simulink model "do_sada"  (R2016b)
settings: Solver=VariableStepAuto  StartTime=0.0  StopTime=10000.0  RelTol=1e-12  AbsTol=1e-9
values from neighbouring files (symbols this model uses):
  d1 = 0.0012    [main.m]
  d2 = 0.0012    [main.m]
  d3 = 0.0012    [main.m]
  h0 = 3    [main.m]
  h10 = 4    [main.m]
  h20 = 4    [main.m]
  h30 = 4    [main.m]
  hmax = 10    [main.m]
  K = acker(Al, Bl, P)    [main.m]
  kr = -1/(Cl * ((Al-Bl*K)\Bl))    [main.m]
  q0 = A * sqrt(h0) / B    [main.m]
  r = 3    [main.m]
  s = 1    [main.m]
  sout = 10e-4    (= 0.001)    [main.m]
settings Model: Creator=Vukan  LastModifiedBy=Vukan

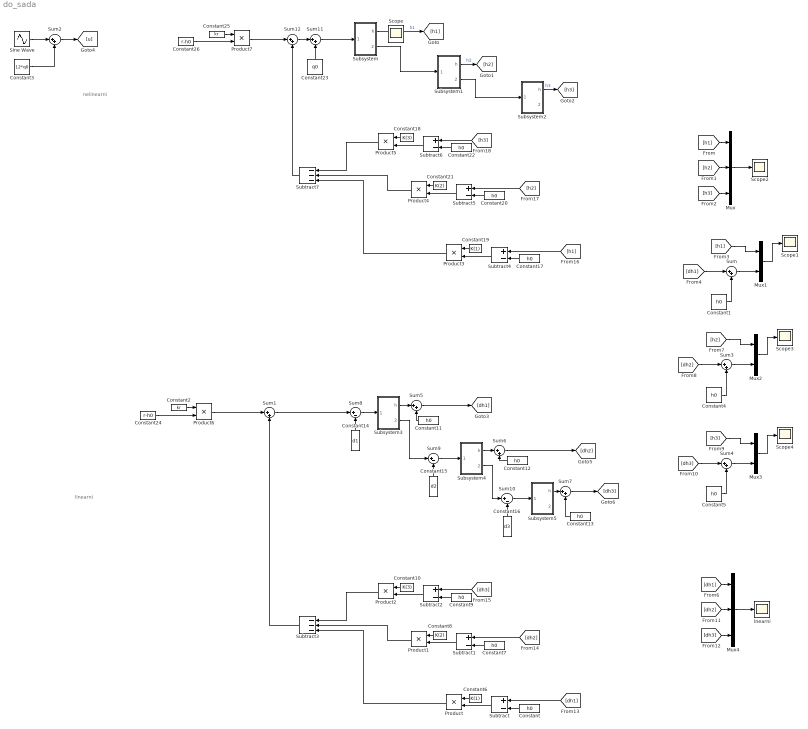
== system do_sada ==
  note: nelinearni
  note: linearni
  Constant{,1,4..5,7,9,11..13,17,20,22} (12 alike) : Constant  Value=h0
  Constant10 : Constant  Value=K(3)
  Constant14 : Constant  Value=d1
  Constant15 : Constant  Value=d2
  Constant16 : Constant  Value=d3
  Constant18 : Constant  Value=K(3)
  Constant19 : Constant  Value=K(1)
  Constant2 : Constant  Value=kr
  Constant21 : Constant  Value=K(2)
  Constant23 : Constant  Value=q0
  Constant24 : Constant  Value=r-h0
  Constant25 : Constant  Value=kr
  Constant26 : Constant  Value=r-h0
  Constant3 : Constant  Value=12*q0
  Constant6 : Constant  Value=K(1)
  Constant8 : Constant  Value=K(2)
  Mux : Mux  Inputs=3
  Mux1 : Mux  Inputs=2
  Mux2 : Mux  Inputs=2
  Mux3 : Mux  Inputs=2
  Mux4 : Mux  Inputs=3
  Product{,1..7} (8 alike) : Product
  Scope{,1..4} (5 alike) : Scope
  Sine Wave : Sin  Amplitude=10*q0  Frequency=0.001*30  SampleTime=0
  Subsystem : Subsystem
  Subsystem1 : Subsystem
  Subsystem2 : Subsystem
  Subsystem3 : Subsystem
  Subsystem4 : Subsystem
  Subsystem5 : Subsystem
  Subtract{,1..2,4..6} (6 alike) : Sum  Inputs=+-
  Subtract3 : Sum  Inputs=---
  Subtract7 : Sum  Inputs=---
  Sum{,1..7,11..12} (10 alike) : Sum  Inputs=|++
  Sum10 : Sum  Inputs=|+-
  Sum8 : Sum  Inputs=|+-
  Sum9 : Sum  Inputs=|+-
  lnearni : Scope
  wires:
  Subsystem/1(h) -> [h1]  "h1"
  Subsystem1/1(h) -> [h2]  "h2"
  Subsystem/2(qout) -> Subsystem1/1(qin)
  Subsystem1/2(qout) -> Subsystem2/1(qin)
  Subsystem2/1(h) -> [h3]  "h3"
  Mux/1 -> Scope2/1
  [h1] -> Mux/1
  [h2] -> Mux/2
  [h3] -> Mux/3
  Mux1/1 -> Scope1/1
  [h1] -> Mux1/1
  [dh1] -> Sum/1
  Sum/1 -> Mux1/2
  Constant1/1 -> Sum/2
  Sum11/1 -> Subsystem/1(qin)
  Sine Wave/1 -> Sum2/1
  Sum2/1 -> [u]
  Constant3/1 -> Sum2/2
  Mux2/1 -> Scope3/1
  [h2] -> Mux2/1
  [dh2] -> Sum3/1
  Sum3/1 -> Mux2/2
  Constant4/1 -> Sum3/2
  Mux3/1 -> Scope4/1
  [h3] -> Mux3/1
  [dh3] -> Sum4/1
  Sum4/1 -> Mux3/2
  Constant5/1 -> Sum4/2
  Constant/1 -> Subtract/2
  Subtract/1 -> Product/2
  Constant6/1 -> Product/1
  Constant7/1 -> Subtract1/2
  Subtract1/1 -> Product1/2
  Constant8/1 -> Product1/1
  Constant9/1 -> Subtract2/2
  Subtract2/1 -> Product2/2
  Constant10/1 -> Product2/1
  Product/1 -> Subtract3/3
  Product1/1 -> Subtract3/2
  Product2/1 -> Subtract3/1
  Mux4/1 -> lnearni/1
  [dh1] -> Mux4/1
  [dh2] -> Mux4/2
  [dh3] -> Mux4/3
  Subsystem3/1(h) -> Sum5/1
  Constant11/1 -> Sum5/2
  Subsystem4/1(h) -> Sum6/1
  Sum6/1 -> [dh2]
  Constant12/1 -> Sum6/2
  Subsystem5/1(h) -> Sum7/1
  Sum7/1 -> [dh3]
  Constant13/1 -> Sum7/2
  Sum5/1 -> [dh1]
  [dh1] -> Subtract/1
  [dh2] -> Subtract1/1
  [dh3] -> Subtract2/1
  Sum8/1 -> Subsystem3/1(delta qin)
  Sum1/1 -> Sum8/1
  Constant14/1 -> Sum8/2
  Constant15/1 -> Sum9/2
  Subsystem3/2(qout) -> Sum9/1
  Sum9/1 -> Subsystem4/1(delta qin)
  Constant16/1 -> Sum10/2
  Sum10/1 -> Subsystem5/1(delta qin)
  Subsystem4/2(qout) -> Sum10/1
  Constant17/1 -> Subtract4/2
  Subtract4/1 -> Product3/2
  Constant19/1 -> Product3/1
  Constant20/1 -> Subtract5/2
  Subtract5/1 -> Product4/2
  Constant21/1 -> Product4/1
  Constant22/1 -> Subtract6/2
  Subtract6/1 -> Product5/2
  Constant18/1 -> Product5/1
  Product3/1 -> Subtract7/3
  Product4/1 -> Subtract7/2
  Product5/1 -> Subtract7/1
  [h1] -> Subtract4/1
  [h2] -> Subtract5/1
  [h3] -> Subtract6/1
  Constant23/1 -> Sum11/2
  Constant24/1 -> Product6/2
  Constant2/1 -> Product6/1
  Product6/1 -> Sum1/1
  Subtract3/1 -> Sum1/2
  Constant26/1 -> Product7/2
  Constant25/1 -> Product7/1
  Sum12/1 -> Sum11/1
  Subtract7/1 -> Sum12/2
  Product7/1 -> Sum12/1

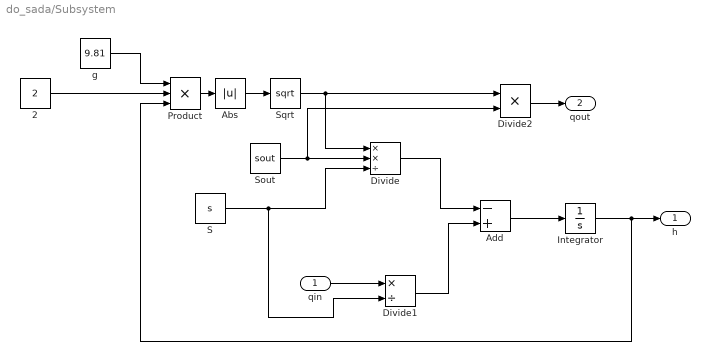
== system do_sada/Subsystem ==
  qin : Inport
  2 : Constant  Value=2
  Abs : Abs
  Add : Sum  Inputs=-+
  Divide : Product  Inputs=**/
  Divide1 : Product  Inputs=*/
  Divide2 : Product  Inputs=**
  Integrator : Integrator  InitialCondition=h10  LimitOutput=on  UpperSaturationLimit=hmax  LowerSaturationLimit=0
  Product : Product  Inputs=3
  "S " : Constant  Value=s
  Sout : Constant  Value=sout
  Sqrt : Sqrt  SaturateOnIntegerOverflow=on
  g : Constant  Value=9.81
  h : Outport
  qout : Outport  Port=2
  wires:
  Sout/1 -> Divide2/2, Divide/2
  "S "/1 -> Divide1/2, Divide/3
  Divide/1 -> Add/1
  qin/1 -> Divide1/1
  Add/1 -> Integrator/1
  g/1 -> Product/1
  Divide1/1 -> Add/2
  Sqrt/1 -> Divide2/1, Divide/1
  2/1 -> Product/2
  Product/1 -> Abs/1
  Abs/1 -> Sqrt/1
  Integrator/1 -> h/1, Product/3
  Divide2/1 -> qout/1

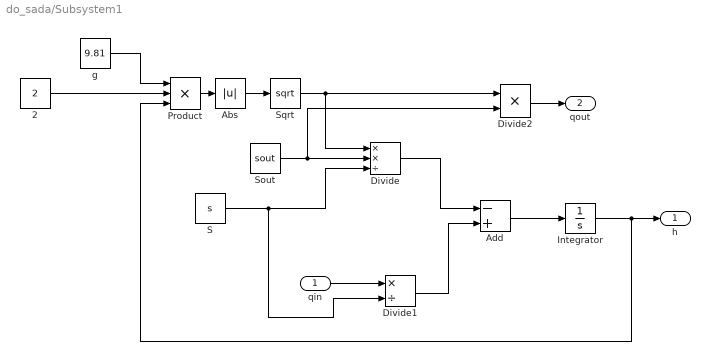
== system do_sada/Subsystem1 ==
  qin : Inport
  2 : Constant  Value=2
  Abs : Abs
  Add : Sum  Inputs=-+
  Divide : Product  Inputs=**/
  Divide1 : Product  Inputs=*/
  Divide2 : Product  Inputs=**
  Integrator : Integrator  InitialCondition=h20  LimitOutput=on  UpperSaturationLimit=hmax  LowerSaturationLimit=0
  Product : Product  Inputs=3
  "S " : Constant  Value=s
  Sout : Constant  Value=sout
  Sqrt : Sqrt  SaturateOnIntegerOverflow=on
  g : Constant  Value=9.81
  h : Outport
  qout : Outport  Port=2
  wires:
  Divide2/1 -> qout/1
  Integrator/1 -> Product/3, h/1
  Abs/1 -> Sqrt/1
  Product/1 -> Abs/1
  2/1 -> Product/2
  Sqrt/1 -> Divide/1, Divide2/1
  Divide1/1 -> Add/2
  g/1 -> Product/1
  Add/1 -> Integrator/1
  qin/1 -> Divide1/1
  Divide/1 -> Add/1
  "S "/1 -> Divide/3, Divide1/2
  Sout/1 -> Divide/2, Divide2/2

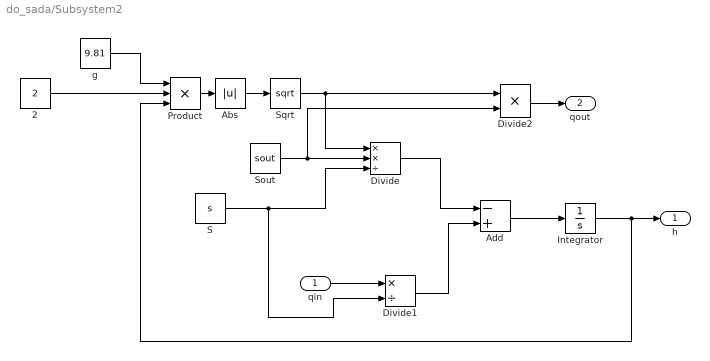
== system do_sada/Subsystem2 ==
  qin : Inport
  2 : Constant  Value=2
  Abs : Abs
  Add : Sum  Inputs=-+
  Divide : Product  Inputs=**/
  Divide1 : Product  Inputs=*/
  Divide2 : Product  Inputs=**
  Integrator : Integrator  InitialCondition=h30  LimitOutput=on  UpperSaturationLimit=hmax  LowerSaturationLimit=0
  Product : Product  Inputs=3
  "S " : Constant  Value=s
  Sout : Constant  Value=sout
  Sqrt : Sqrt  SaturateOnIntegerOverflow=on
  g : Constant  Value=9.81
  h : Outport
  qout : Outport  Port=2
  wires:
  Sout/1 -> Divide2/2, Divide/2
  "S "/1 -> Divide1/2, Divide/3
  Divide/1 -> Add/1
  qin/1 -> Divide1/1
  Add/1 -> Integrator/1
  g/1 -> Product/1
  Divide1/1 -> Add/2
  Sqrt/1 -> Divide2/1, Divide/1
  2/1 -> Product/2
  Product/1 -> Abs/1
  Abs/1 -> Sqrt/1
  Integrator/1 -> h/1, Product/3
  Divide2/1 -> qout/1

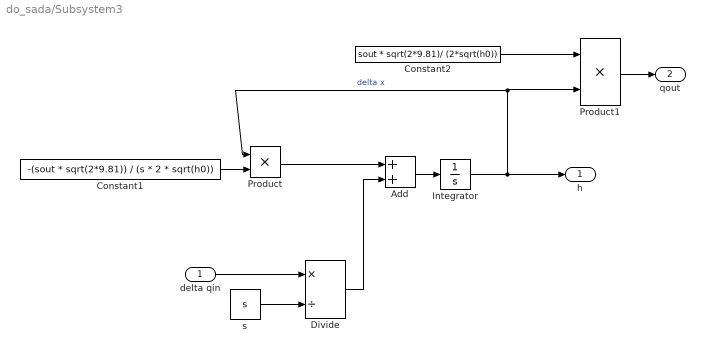
== system do_sada/Subsystem3 ==
  delta qin : Inport
  Add : Sum
  Constant1 : Constant  Value=-(sout * sqrt(2*9.81)) / (s * 2 * sqrt(h0))
  Constant2 : Constant  Value=sout * sqrt(2*9.81)/ (2*sqrt(h0))
  Divide : Product  Inputs=*/
  Integrator : Integrator  InitialCondition=1
  Product : Product
  Product1 : Product
  s : Constant  Value=s
  h : Outport
  qout : Outport  Port=2
  wires:
  Integrator/1 -> h/1, Product1/2, Product/1  "delta x"
  Product/1 -> Add/1
  Add/1 -> Integrator/1
  delta qin/1 -> Divide/1
  Product1/1 -> qout/1
  Divide/1 -> Add/2
  Constant2/1 -> Product1/1
  Constant1/1 -> Product/2
  s/1 -> Divide/2

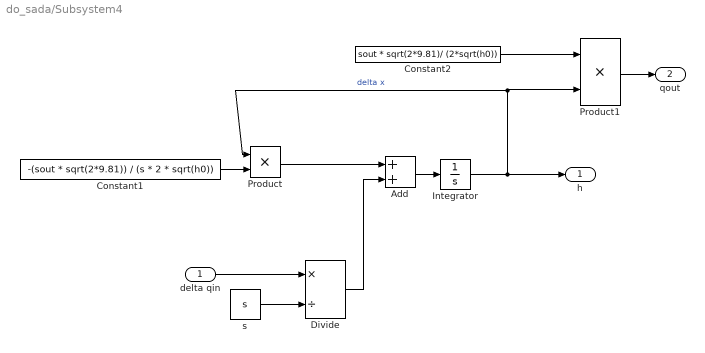
== system do_sada/Subsystem4 ==
  delta qin : Inport
  Add : Sum
  Constant1 : Constant  Value=-(sout * sqrt(2*9.81)) / (s * 2 * sqrt(h0))
  Constant2 : Constant  Value=sout * sqrt(2*9.81)/ (2*sqrt(h0))
  Divide : Product  Inputs=*/
  Integrator : Integrator  InitialCondition=1
  Product : Product
  Product1 : Product
  s : Constant  Value=s
  h : Outport
  qout : Outport  Port=2
  wires:
  s/1 -> Divide/2
  Constant1/1 -> Product/2
  Constant2/1 -> Product1/1
  Divide/1 -> Add/2
  Product1/1 -> qout/1
  delta qin/1 -> Divide/1
  Add/1 -> Integrator/1
  Product/1 -> Add/1
  Integrator/1 -> Product/1, Product1/2, h/1  "delta x"

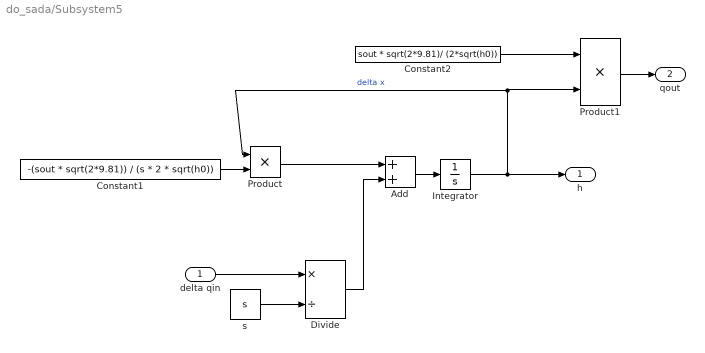
== system do_sada/Subsystem5 ==
  delta qin : Inport
  Add : Sum
  Constant1 : Constant  Value=-(sout * sqrt(2*9.81)) / (s * 2 * sqrt(h0))
  Constant2 : Constant  Value=sout * sqrt(2*9.81)/ (2*sqrt(h0))
  Divide : Product  Inputs=*/
  Integrator : Integrator  InitialCondition=1
  Product : Product
  Product1 : Product
  s : Constant  Value=s
  h : Outport
  qout : Outport  Port=2
  wires:
  Integrator/1 -> h/1, Product1/2, Product/1  "delta x"
  Product/1 -> Add/1
  Add/1 -> Integrator/1
  delta qin/1 -> Divide/1
  Product1/1 -> qout/1
  Divide/1 -> Add/2
  Constant2/1 -> Product1/1
  Constant1/1 -> Product/2
  s/1 -> Divide/2
